simulink model "DC_LQI"  (R2015a)
settings: Solver=ode45  StartTime=0.0  StopTime=80.0  RelTol=1e-3
values from neighbouring files (symbols this model uses):
  A = [-50 -2833.3;0.85 0]    [DC_PID_IMC.m]    (also in data.mat = [-50  -2833.3; 0.85  0])
  b = [333.3; 0]    [DC_PID_IMC.m]    (also in data.mat = [333.3 0])
  c = [0 1]    [DC_PID_IMC.m]    (also in data.mat)
  D = [1 1]    [DC_PID_IMC.m]    (also in data.mat)
  Jw = [0 1]    [DC_PID_IMC.m]    (also in data.mat)
  k1 = [0.0004 0.0208]    [DC_PID_IMC.m]    (also in data.mat)
  k2 = [0.9996]    [DC_PID_IMC.m]    (also in data.mat = 0.9996)
undefined symbols (not defined in the file or in its folder): sigbuilder_block
settings Model: Creator=yusuke  LastModifiedBy=yusuke

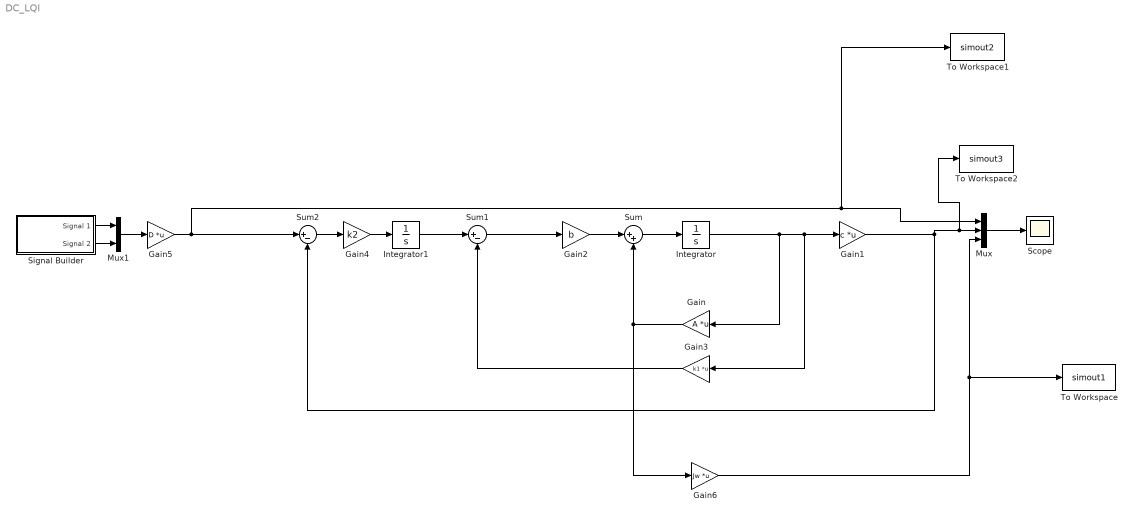
== system DC_LQI ==
  Gain : Gain  Gain=A  Multiplication=Matrix(K*u) (u vector)
  Gain1 : Gain  Gain=c  Multiplication=Matrix(K*u) (u vector)
  Gain2 : Gain  Gain=b
  Gain3 : Gain  Gain=k1  Multiplication=Matrix(K*u) (u vector)
  Gain4 : Gain  Gain=k2
  Gain5 : Gain  Gain=D  Multiplication=Matrix(K*u) (u vector)
  Gain6 : Gain  Gain=Jw  Multiplication=Matrix(K*u) (u vector)
  Integrator : Integrator
  Integrator1 : Integrator
  Mux : Mux  Inputs=3
  Mux1 : Mux  Inputs=2
  Scope : Scope
      settings: TimeRange=15  YMin=0  YMax=2
  Signal Builder : Subsystem  Tag=STV Subsys  LoadFcn=sigbuilder_block('load');  StartFcn=sigbuilder_block('start');  StopFcn=sigbuilder_block('stop');  ClipboardFcn=sigbuilder_block('clipboard');  mask(Sigbuilder block){}
      mask help: Simulink:masks:SigbuilderBlock_MD
      mask init:
      | if ~strcmp(get_param(bdroot(gcbh),'SimulationStatus'),'stopped') tuvar = sigbuilder_block('maskInit'); end
      settings: CopyFcn=sigbuilder_block('copy');  DeleteFcn=sigbuilder_block('delete');  ModelCloseFcn=sigbuilder_block('modelClose');  PreSaveFcn=sigbuilder_block('preSave');  PauseFcn=sigbuilder_block('pause');  ContinueFcn=sigbuilder_block('continue');  NameChangeFcn=sigbuilder_block('namechange');  OpenFcn=sigbuilder_block('open',[437.6 199.2 550.4 400 ]);  CloseFcn=sigbuilder_block('close');
      mask Display: plot(0, 0, 100, 100,[2, 2, 32, 32, 2], [68, 8, 8, 68, 68],[32, 2], [38, 38], [32, 19, 2],[53, 60, 44], [32, 17, 17, 2],[16, 16, 31, 31]);txt = getActiveGroup(gcbh);text(2, 100, txt,'verticalAlignment', 'top');
  Sum : Sum  Inputs=|++
  Sum1 : Sum  Inputs=|+-
  Sum2 : Sum  Inputs=|+-
  To Workspace : ToWorkspace  VariableName=simout1  SaveFormat=Structure With Time  SampleTime=-1
  To Workspace1 : ToWorkspace  VariableName=simout2  SaveFormat=Structure With Time  SampleTime=-1
  To Workspace2 : ToWorkspace  VariableName=simout3  SaveFormat=Structure With Time  SampleTime=-1
  wires:
  Integrator/1 -> Gain/1, Gain3/1, Gain1/1
  Gain/1 -> Sum/2, Gain6/1
  Gain2/1 -> Sum/1
  Sum/1 -> Integrator/1
  Gain1/1 -> Sum2/2, To Workspace2/1, Mux/2
  Sum1/1 -> Gain2/1
  Gain3/1 -> Sum1/2
  Integrator1/1 -> Sum1/1
  Gain4/1 -> Integrator1/1
  Sum2/1 -> Gain4/1
  Gain5/1 -> To Workspace1/1, Mux/1, Sum2/1
  Mux/1 -> Scope/1
  Signal Builder/2(Signal 2) -> Mux1/2
  Mux1/1 -> Gain5/1
  Signal Builder/1(Signal 1) -> Mux1/1
  Gain6/1 -> To Workspace/1, Mux/3

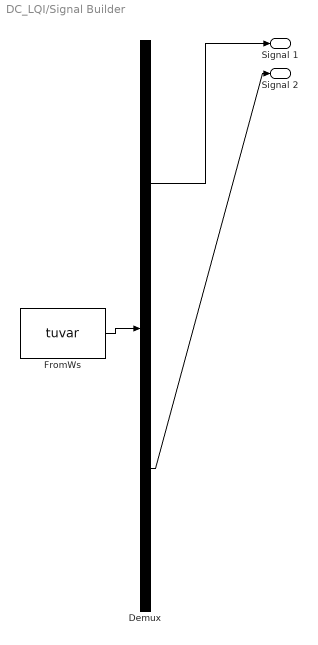
== system DC_LQI/Signal Builder ==
  Demux : Demux  Tag=STV Demux  Outputs=2
  FromWs : FromWorkspace  Tag=STV FromWs  VariableName=tuvar  SampleTime=0
      SigBuilderData=|
      | common.afterFinalStr = 'Extrapolate'
      | common.sampleTime = 0
      | dataSet.timeRange = [0 80]
      | dataSet.name = 'Group 1'
      | sbobj.Groups.Name = 'Group 1'
      | sbobj.Groups.Signals(1).Name = 'Signal 1'
      | sbobj.Groups.Signals(1).XData = [0 20 20 80]
      | sbobj.Groups.Signals(1).YData = [500 500 0 0]
      | sbobj.Groups.Signals(2).Name = 'Signal 2'
      | sbobj.Groups.Signals(2).XData = [0 40 40 60 60 80]
      | sbobj.Groups.Signals(2).YData = [0 0 -500 -500 0 0]
      | sbobj.Groups.TimeRange = [0 80]
  Signal 1 : Outport  Tag=STV Outport
  Signal 2 : Outport  Tag=STV Outport  Port=2
  wires:
  Demux/1 -> Signal 1/1
  FromWs/1 -> Demux/1
  Demux/2 -> Signal 2/1
